simulink model "GsqRealHighVolt"  (R2015a)
settings: configuration reference "SIMULATION_CONFIGURATION" (kept outside this file)
settings Model: CovSFcnEnable=off  Creator=moritz  LastModifiedBy=moritz
settings ConfigSetRef: SourceLocation=Base Workspace

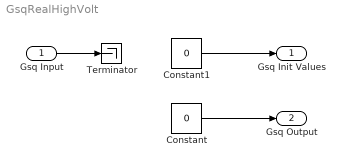
== system GsqRealHighVolt ==
  Gsq Input : Inport  OutDataTypeStr=Bus: GSQ_INPUT_BUS  BusOutputAsStruct=on
  Constant : Constant  Value=0  OutDataTypeStr=Bus: GSQ_OUTPUT_BUS
  Constant1 : Constant  Value=0  OutDataTypeStr=Bus: GSQ_INPUT_BUS
  Terminator : Terminator
  Gsq Init Values : Outport  OutDataTypeStr=Bus: GSQ_INPUT_BUS  BusOutputAsStruct=on
  Gsq Output : Outport  Port=2  OutDataTypeStr=Bus: GSQ_OUTPUT_BUS  BusOutputAsStruct=on
  wires:
  Constant/1 -> Gsq Output/1
  Gsq Input/1 -> Terminator/1
  Constant1/1 -> Gsq Init Values/1
